simulink model "lab_1_2_contr"  (R2023b)
settings: Solver=FixedStepAuto  StartTime=0.0  StopTime=10.0  FixedStep=0.0001  RelTol=1e-3
undefined symbols (not defined in the file): a_0, a_1, a_2, b_0, b_1, b_2
settings Model: Creator=nsukh  LastModifiedBy=nsukh

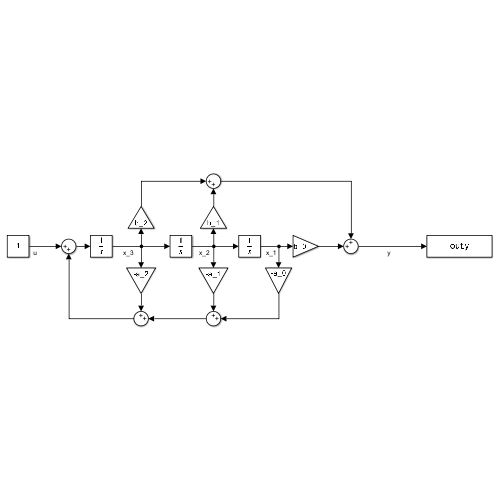
[thumbnail: Simulink's stored preview of the top-level diagram]
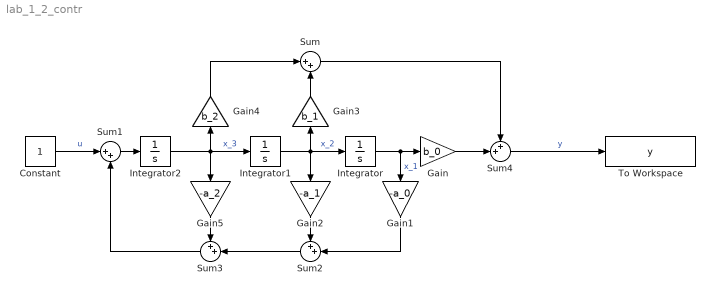
== system lab_1_2_contr ==
  Constant : Constant  SampleTime=-1
  Gain : Gain  Gain=b_0
  Gain1 : Gain  Gain=-a_0
  Gain2 : Gain  Gain=-a_1
  Gain3 : Gain  Gain=b_1
  Gain4 : Gain  Gain=b_2
  Gain5 : Gain  Gain=-a_2
  Integrator : Integrator
  Integrator1 : Integrator
  Integrator2 : Integrator
  Sum : Sum  Inputs=|++
  Sum1 : Sum  Inputs=|++
  Sum2 : Sum  Inputs=++|
  Sum3 : Sum  Inputs=++|
  Sum4 : Sum  Inputs=++|
  To Workspace : ToWorkspace  VariableName=y  SaveFormat=Timeseries  SampleTime=-1
  wires:
  Sum4/1 -> To Workspace/1  "y"
  Sum/1 -> Sum4/1
  Integrator/1 -> Gain1/1, Gain/1  "x_1"
  Integrator1/1 -> Integrator/1, Gain3/1, Gain2/1  "x_2"
  Gain3/1 -> Sum/2
  Gain4/1 -> Sum/1
  Integrator2/1 -> Gain4/1, Gain5/1, Integrator1/1  "x_3"
  Sum3/1 -> Sum1/2
  Sum1/1 -> Integrator2/1
  Constant/1 -> Sum1/1  "u"
  Gain1/1 -> Sum2/2
  Gain2/1 -> Sum2/1
  Gain5/1 -> Sum3/1
  Sum2/1 -> Sum3/2
  Gain/1 -> Sum4/2
